simulink model "Single_Tank"  (R2018b)
settings: Solver=VariableStepAuto  StartTime=0.0  StopTime=100  RelTol=1e-3
settings Model: Creator=daiba  LastModifiedBy=daiba

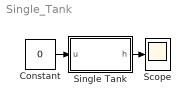
== system Single_Tank ==
  Constant : Constant  Value=0
  Scope : Scope
  Single Tank : Subsystem  mask{AA=10, a=5, k=0.1, Cd=0.05, g=9.81, h_zero=1}
      mask prompts: AA "Tiet dien ngang bon chua"; a "Tiet dien van xa"; k "He so ti le cong suat may bom"; Cd "He so xa"; g "Gia toc trong truong"; h_zero "Muc nuoc ban dau"
  wires:
  Constant/1 -> Single Tank/1(u)
  Single Tank/1(h) -> Scope/1

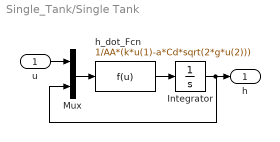
== system Single_Tank/Single Tank ==
  u : Inport
  Integrator : Integrator  InitialCondition=h_zero
  Mux : Mux  Inputs=2
  h_dot_Fcn : Fcn  Expr=1/AA*(k*u(1)-a*Cd*sqrt(2*g*u(2)))
  h : Outport
  wires:
  Mux/1 -> h_dot_Fcn/1
  u/1 -> Mux/1
  h_dot_Fcn/1 -> Integrator/1
  Integrator/1 -> Mux/2, h/1
